simulink model "problem3"  (R2020a)
settings: Solver=VariableStepAuto  StartTime=0.0  StopTime=10.0  RelTol=1e-3
model workspace (MAT data in the model file):
  K1 = 0.579
  K2 = 0.1584
settings Model: Creator=USER  LastModifiedBy=USER

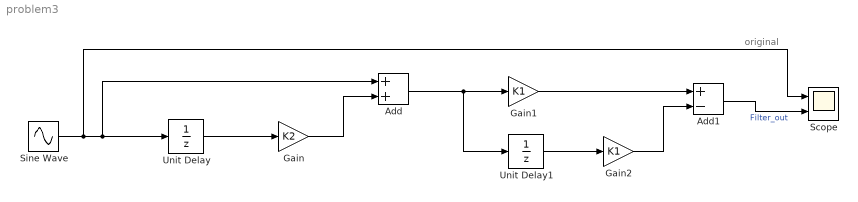
== system problem3 ==
  note: original
  Add : Sum
  Add1 : Sum  Inputs=+-
  Gain : Gain  Gain=K2
  Gain1 : Gain  Gain=K1
  Gain2 : Gain  Gain=K1
  Scope : Scope  NumInputPorts=2
  Sine Wave : Sin  Frequency=100*2*pi  SampleTime=1/5000
  Unit Delay : UnitDelay  SampleTime=-1  HasFrameUpgradeWarning=on
  Unit Delay1 : UnitDelay  SampleTime=-1  HasFrameUpgradeWarning=on
  wires:
  Add1/1 -> Scope/2  "Filter_out"
  Unit Delay1/1 -> Gain2/1
  Gain2/1 -> Add1/2
  Unit Delay/1 -> Gain/1
  Gain1/1 -> Add1/1
  Add/1 -> Unit Delay1/1, Gain1/1
  Sine Wave/1 -> Scope/1, Add/1, Unit Delay/1
  Gain/1 -> Add/2
